simulink model "pidControl"  (R2019b)
settings: Solver=VariableStepAuto  StartTime=0.0  StopTime=10.0  RelTol=1e-3
undefined symbols (not defined in the file or in its folder): calib
libraries: arduinolib x10, simulink x4, dspstat3 x3
settings Model: Creator=Victor  LastModifiedBy=covasanvictor

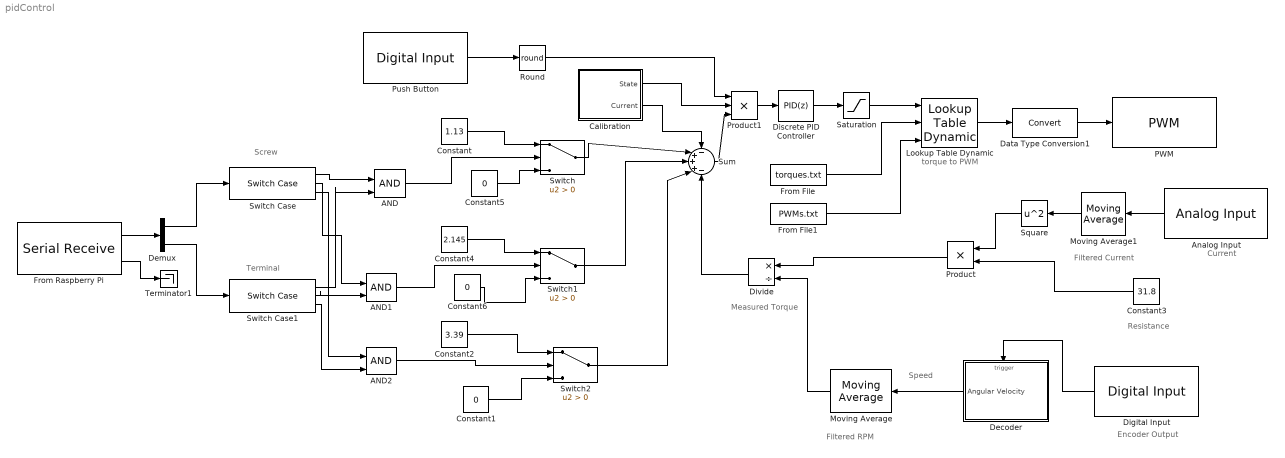
== system pidControl ==
  note: Filtered Current
  note: Filtered RPM
  note: Encoder Output
  note: Measured
      | Torque
  note: Speed
  note: Screw
  note: torque to PWM
  note: Current
  note: Resistance
  note: Terminal
  AND : Logic  IconShape=distinctive  AllPortsSameDT=off  OutDataTypeStr=boolean
  AND1 : Logic  IconShape=distinctive  AllPortsSameDT=off  OutDataTypeStr=boolean
  AND2 : Logic  IconShape=distinctive  AllPortsSameDT=off  OutDataTypeStr=boolean
  Analog Input : arduinolib/Analog Input  pinNumber=0  ReadResultsOnly=off  ConversionTriggerSource=Software  ExternalTriggerType=uint32( 0 )  OutputDataType=uint16  EnableConversionCompleteNotify=off  EnableOuputStatus=off  SampleTime=-1  blockPlatform=arduino
  "Calibration " : Subsystem
  Constant : Constant  Value=1.13
  Constant1 : Constant  Value=0
  Constant2 : Constant  Value=3.39
  Constant3 : Constant  Value=31.8
  Constant4 : Constant  Value=2.145
  Constant5 : Constant  Value=0
  Constant6 : Constant  Value=0
  Data Type Conversion1 : DataTypeConversion  OutMin=[0]  OutMax=[255]
  "Decoder " : Subsystem
  Demux : Demux  Outputs=2
  Digital Input : arduinolib/Digital Input  pinNumber=2  SampleTime=-1  blockPlatform=arduino
      settings: SourceProductName=Simulink Support Package for Arduino Hardware
  Discrete PID Controller : simulink/Continuous/PID Controller  Controller=PID  Form=Parallel  TimeDomain=Discrete-time  SampleTime=-1  IntegratorMethod=Forward Euler  FilterMethod=Forward Euler  ControllerParametersSource=internal  P=10  I=0.1  D=0  UseFilter=on  N=100  TunerSelectOption=Transfer Function Based (PID Tuner App)  InitialConditionSource=internal  InitialConditionForIntegrator=0  InitialConditionForFilter=0  DifferentiatorICPrevScaledInput=0  ExternalReset=none  TrackingMode=off  Kt=1  LimitOutput=off  UpperSaturationLimit=inf  LowerSaturationLimit=-inf  LinearizeAsGain=off  AntiWindupMode=none  Kb=1  POutMin=[]  POutMax=[]  IOutMin=[]  IOutMax=[]  DOutMin=[]  DOutMax=[]  NOutMin=[]  NOutMax=[]  SumOutMin=[]  SumOutMax=[]  SaturationOutMin=[]  SaturationOutMax=[]  PParamMin=[]  PParamMax=[]  IParamMin=[]  IParamMax=[]  DParamMin=[]  DParamMax=[]  NParamMin=[]  NParamMax=[]  KbParamMin=[]  KbParamMax=[]  KtParamMin=[]  KtParamMax=[]  KbOutMin=[]  KbOutMax=[]  KtOutMin=[]  KtOutMax=[]  IntegratorOutMin=[]  IntegratorOutMax=[]  FilterOutMin=[]  FilterOutMax=[]  SumI1OutMin=[]  SumI1OutMax=[]  SumI2OutMin=[]  SumI2OutMax=[]  SumI3OutMin=[]  SumI3OutMax=[]  SumI4OutMin=[]  SumI4OutMax=[]  SumDOutMin=[]  SumDOutMax=[]  DifferentiatorOutMin=[]  DifferentiatorOutMax=[]  FilterDiffOutCoefMin=[]  FilterDiffOutCoefMax=[]  ReciprocalOutMin=[]  ReciprocalOutMax=[]  SumDenOutMin=[]  SumDenOutMax=[]  SumNumOutMin=[]  SumNumOutMax=[]  DivideOutMin=[]  DivideOutMax=[]  IntegratorContinuousStateAttributes=''  IntegratorStateMustResolveToSignalObject=off  IntegratorRTWStateStorageClass=Auto  FilterContinuousStateAttributes=''  FilterStateMustResolveToSignalObject=off  FilterRTWStateStorageClass=Auto  ParallelPVariant=InternalParameters  IdealPVariant=Disabled  IVariant=InternalParameters  DVariant=InternalParameters  IntegratorVariant=Discrete  SatVariant=Disabled  AWVariant=Passthrough  PCopyVariant=Disabled  TRVariant=Disabled  FdbkBlocksVariant=Forward  IdealPFdbkVariant=Disabled  SatFdbkVariant=Disabled  DerivativeFilterVariant=ForwardEulerFilter  NVariant=InternalParameters  NCopyVariant=Disabled  FilterICVariant=InternalICsFilter  IntegratorICVariant=InternalICs  ExternalResetVariant=Disabled  TRSumVariant=Passthrough  SumFdbkVariant=Disabled  SumVariant=Sum_PID
  Divide : Product  Inputs=*/
  From File : FromFile  FileName=torques.txt  SampleTime=0
  From File1 : FromFile  FileName=PWMs.txt  SampleTime=0
  "From Raspberry Pi " : arduinolib/Serial Receive  isARMArch=off  portNumber=0  DataType=uint8  Datalength=2  SampleTime=0.1  showOutStatus=on  blockPlatform=arduino
      settings: SourceProductName=Simulink Support Package for Arduino Hardware  SourceProductBaseCode=ARDUINO
  Lookup Table Dynamic : simulink/Lookup Tables/Lookup Table Dynamic  LookUpMeth=Interpolation-Use End Values  OutDataType=fixdt('double')  OutScaling=[]  OutputDataTypeScalingMode=Specify via dialog  OutDataTypeStr=double  DoSatur=off
  Moving Average : dspstat3/Moving Average  Method=Sliding window  ForgettingFactorPort=off  SpecifyWindowLength=on  WindowLength=4  ForgettingFactor=0.9  SimulateUsing=Code generation
  Moving Average1 : dspstat3/Moving Average  Method=Sliding window  ForgettingFactorPort=off  SpecifyWindowLength=on  WindowLength=4  ForgettingFactor=0.9  SimulateUsing=Code generation
  PWM : arduinolib/PWM  pinNumber=6  EnableInputFrequency=off  InitialFrequency=2000  InitialDutyCycle=0  NotificationType=None  blockPlatform=arduino
  Product : Product
  Product1 : Product  Inputs=3
  "Push Button " : arduinolib/Digital Input  pinNumber=8  SampleTime=-1  blockPlatform=arduino
      settings: SourceProductName=Simulink Support Package for Arduino Hardware
  Round : Rounding  Operator=round
  Saturation : Saturate
  Square : Math  Operator=square  SignedPower=off  SaturateOnIntegerOverflow=on
  Sum : Sum  Inputs=-+++-
  Switch : Switch  Criteria=u2 > Threshold
  Switch Case : SwitchCase  CaseConditions={1, 2, 3}  ShowDefaultCase=off
  Switch Case1 : SwitchCase  CaseConditions={1, 2, 3}  ShowDefaultCase=off
  Switch1 : Switch  Criteria=u2 > Threshold
  Switch2 : Switch  Criteria=u2 > Threshold
  Terminator1 : Terminator
  wires:
  Constant3/1 -> Product/2
  Square/1 -> Product/1
  "Decoder "/1("Angular Velocity ") -> Moving Average/1
  Product/1 -> Divide/1
  Discrete PID Controller/1 -> Saturation/1
  Constant/1 -> Switch/1
  Saturation/1 -> Lookup Table Dynamic/1
  From File/1 -> Lookup Table Dynamic/2
  From File1/1 -> Lookup Table Dynamic/3
  Switch Case/1 -> AND/1
  Switch Case1/1 -> AND/2
  AND/1 -> Switch/2
  Moving Average/1 -> Divide/2
  Constant5/1 -> Switch/3
  Switch Case1/2 -> AND1/2
  Switch Case/2 -> AND1/1
  Constant6/1 -> Switch1/3
  Constant4/1 -> Switch1/1
  AND1/1 -> Switch1/2
  Switch Case/3 -> AND2/1
  Switch Case1/3 -> AND2/2
  Constant1/1 -> Switch2/3
  Constant2/1 -> Switch2/1
  AND2/1 -> Switch2/2
  "From Raspberry Pi "/1 -> Demux/1
  Demux/1 -> Switch Case/1
  Demux/2 -> Switch Case1/1
  "From Raspberry Pi "/2 -> Terminator1/1
  Lookup Table Dynamic/1 -> Data Type Conversion1/1
  Data Type Conversion1/1 -> PWM/1
  Digital Input/1 -> "Decoder "/Trigger
  Product1/1 -> Discrete PID Controller/1
  "Calibration "/1(State) -> Product1/2
  Sum/1 -> Product1/3
  "Push Button "/1 -> Round/1
  Round/1 -> Product1/1
  Divide/1 -> Sum/5
  Switch2/1 -> Sum/4
  Switch1/1 -> Sum/3
  Switch/1 -> Sum/2
  "Calibration "/2("Current ") -> Sum/1
  Moving Average1/1 -> Square/1
  Analog Input/1 -> Moving Average1/1

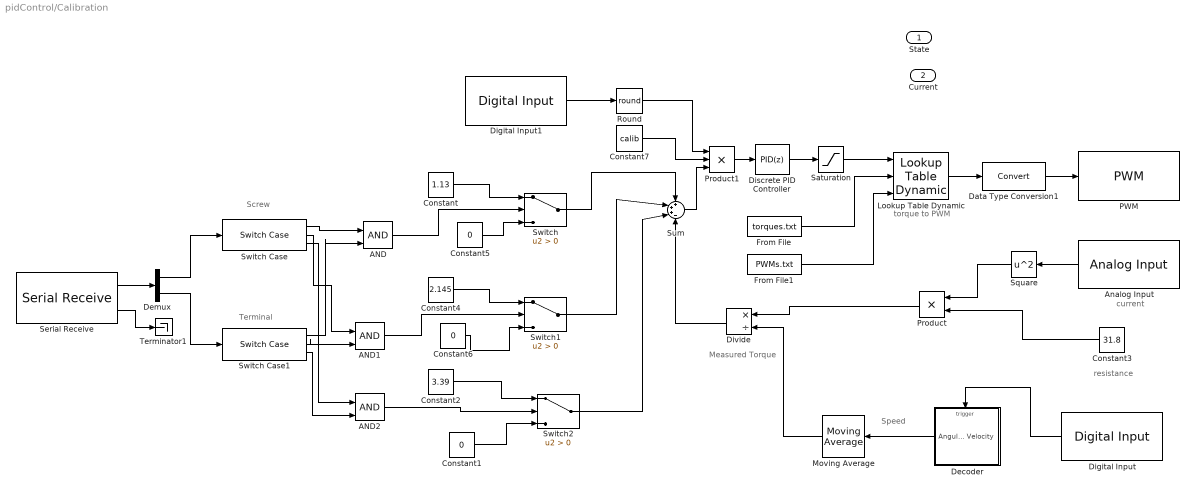
== system pidControl/Calibration  ==
  note: Terminal
  note: current
  note: resistance
  note: Screw
  note: torque to PWM
  note: Speed
  note: Measured
      | Torque
  AND : Logic  IconShape=distinctive  AllPortsSameDT=off  OutDataTypeStr=boolean
  AND1 : Logic  IconShape=distinctive  AllPortsSameDT=off  OutDataTypeStr=boolean
  AND2 : Logic  IconShape=distinctive  AllPortsSameDT=off  OutDataTypeStr=boolean
  Analog Input : arduinolib/Analog Input  pinNumber=0  ReadResultsOnly=off  ConversionTriggerSource=Software  ExternalTriggerType=uint32( 0 )  OutputDataType=uint16  EnableConversionCompleteNotify=off  EnableOuputStatus=off  SampleTime=-1  blockPlatform=arduino
  Constant : Constant  Value=1.13
  Constant1 : Constant  Value=0
  Constant2 : Constant  Value=3.39
  Constant3 : Constant  Value=31.8
  Constant4 : Constant  Value=2.145
  Constant5 : Constant  Value=0
  Constant6 : Constant  Value=0
  Constant7 : Constant  Value=calib
  Data Type Conversion1 : DataTypeConversion  OutMin=[0]  OutMax=[255]
  "Decoder " : Subsystem
  Demux : Demux  Outputs=2
  Digital Input : arduinolib/Digital Input  pinNumber=2  SampleTime=-1  blockPlatform=arduino
      settings: SourceProductName=Simulink Support Package for Arduino Hardware
  Digital Input1 : arduinolib/Digital Input  pinNumber=8  SampleTime=-1  blockPlatform=arduino
      settings: SourceProductName=Simulink Support Package for Arduino Hardware
  Discrete PID Controller : simulink/Continuous/PID Controller  Controller=PID  Form=Parallel  TimeDomain=Discrete-time  SampleTime=-1  IntegratorMethod=Forward Euler  FilterMethod=Forward Euler  ControllerParametersSource=internal  P=10  I=0.1  D=0  UseFilter=on  N=100  TunerSelectOption=Transfer Function Based (PID Tuner App)  InitialConditionSource=internal  InitialConditionForIntegrator=0  InitialConditionForFilter=0  DifferentiatorICPrevScaledInput=0  ExternalReset=none  TrackingMode=off  Kt=1  LimitOutput=off  UpperSaturationLimit=inf  LowerSaturationLimit=-inf  LinearizeAsGain=off  AntiWindupMode=none  Kb=1  POutMin=[]  POutMax=[]  IOutMin=[]  IOutMax=[]  DOutMin=[]  DOutMax=[]  NOutMin=[]  NOutMax=[]  SumOutMin=[]  SumOutMax=[]  SaturationOutMin=[]  SaturationOutMax=[]  PParamMin=[]  PParamMax=[]  IParamMin=[]  IParamMax=[]  DParamMin=[]  DParamMax=[]  NParamMin=[]  NParamMax=[]  KbParamMin=[]  KbParamMax=[]  KtParamMin=[]  KtParamMax=[]  KbOutMin=[]  KbOutMax=[]  KtOutMin=[]  KtOutMax=[]  IntegratorOutMin=[]  IntegratorOutMax=[]  FilterOutMin=[]  FilterOutMax=[]  SumI1OutMin=[]  SumI1OutMax=[]  SumI2OutMin=[]  SumI2OutMax=[]  SumI3OutMin=[]  SumI3OutMax=[]  SumI4OutMin=[]  SumI4OutMax=[]  SumDOutMin=[]  SumDOutMax=[]  DifferentiatorOutMin=[]  DifferentiatorOutMax=[]  FilterDiffOutCoefMin=[]  FilterDiffOutCoefMax=[]  ReciprocalOutMin=[]  ReciprocalOutMax=[]  SumDenOutMin=[]  SumDenOutMax=[]  SumNumOutMin=[]  SumNumOutMax=[]  DivideOutMin=[]  DivideOutMax=[]  IntegratorContinuousStateAttributes=''  IntegratorStateMustResolveToSignalObject=off  IntegratorRTWStateStorageClass=Auto  FilterContinuousStateAttributes=''  FilterStateMustResolveToSignalObject=off  FilterRTWStateStorageClass=Auto  ParallelPVariant=InternalParameters  IdealPVariant=Disabled  IVariant=InternalParameters  DVariant=InternalParameters  IntegratorVariant=Discrete  SatVariant=Disabled  AWVariant=Passthrough  PCopyVariant=Disabled  TRVariant=Disabled  FdbkBlocksVariant=Forward  IdealPFdbkVariant=Disabled  SatFdbkVariant=Disabled  DerivativeFilterVariant=ForwardEulerFilter  NVariant=InternalParameters  NCopyVariant=Disabled  FilterICVariant=InternalICsFilter  IntegratorICVariant=InternalICs  ExternalResetVariant=Disabled  TRSumVariant=Passthrough  SumFdbkVariant=Disabled  SumVariant=Sum_PID
  Divide : Product  Inputs=*/
  From File : FromFile  FileName=torques.txt  SampleTime=0
  From File1 : FromFile  FileName=PWMs.txt  SampleTime=0
  Lookup Table Dynamic : simulink/Lookup Tables/Lookup Table Dynamic  LookUpMeth=Interpolation-Use End Values  OutDataType=fixdt('double')  OutScaling=[]  OutputDataTypeScalingMode=Specify via dialog  OutDataTypeStr=double  DoSatur=off
  Moving Average : dspstat3/Moving Average  Method=Sliding window  ForgettingFactorPort=off  SpecifyWindowLength=on  WindowLength=4  ForgettingFactor=0.9  SimulateUsing=Code generation
  PWM : arduinolib/PWM  pinNumber=6  EnableInputFrequency=off  InitialFrequency=2000  InitialDutyCycle=0  NotificationType=None  blockPlatform=arduino
  Product : Product
  Product1 : Product  Inputs=3
  Round : Rounding  Operator=round
  Saturation : Saturate
  Serial Receive : arduinolib/Serial Receive  isARMArch=off  portNumber=0  DataType=uint8  Datalength=2  SampleTime=0.1  showOutStatus=on  blockPlatform=arduino
      settings: SourceProductName=Simulink Support Package for Arduino Hardware  SourceProductBaseCode=ARDUINO
  Square : Math  Operator=square  SignedPower=off  SaturateOnIntegerOverflow=on
  Sum : Sum  Inputs=+++-
  Switch : Switch  Criteria=u2 > Threshold
  Switch Case : SwitchCase  CaseConditions={1, 2, 3}  ShowDefaultCase=off
  Switch Case1 : SwitchCase  CaseConditions={1, 2, 3}  ShowDefaultCase=off
  Switch1 : Switch  Criteria=u2 > Threshold
  Switch2 : Switch  Criteria=u2 > Threshold
  Terminator1 : Terminator
  State : Outport
  "Current " : Outport  Port=2
  wires:
  Data Type Conversion1/1 -> PWM/1
  Product1/1 -> Discrete PID Controller/1
  Sum/1 -> Product1/3
  Analog Input/1 -> Square/1
  AND2/1 -> Switch2/2
  "Decoder "/1("Angular Velocity ") -> Moving Average/1
  Lookup Table Dynamic/1 -> Data Type Conversion1/1
  Digital Input1/1 -> Round/1
  Switch/1 -> Sum/1
  Serial Receive/2 -> Terminator1/1
  From File1/1 -> Lookup Table Dynamic/3
  Demux/1 -> Switch Case/1
  Square/1 -> Product/1
  Switch Case/3 -> AND2/1
  Constant1/1 -> Switch2/3
  AND1/1 -> Switch1/2
  AND/1 -> Switch/2
  Switch Case1/1 -> AND/2
  Constant7/1 -> Product1/2
  Round/1 -> Product1/1
  Discrete PID Controller/1 -> Saturation/1
  Constant/1 -> Switch/1
  Constant5/1 -> Switch/3
  Switch2/1 -> Sum/3
  Digital Input/1 -> "Decoder "/Trigger
  Saturation/1 -> Lookup Table Dynamic/1
  Switch Case/1 -> AND/1
  Switch Case1/3 -> AND2/2
  Moving Average/1 -> Divide/2
  Demux/2 -> Switch Case1/1
  Constant3/1 -> Product/2
  Constant4/1 -> Switch1/1
  Switch1/1 -> Sum/2
  Divide/1 -> Sum/4
  Constant2/1 -> Switch2/1
  Constant6/1 -> Switch1/3
  Product/1 -> Divide/1
  Switch Case1/2 -> AND1/2
  Serial Receive/1 -> Demux/1
  From File/1 -> Lookup Table Dynamic/2
  Switch Case/2 -> AND1/1

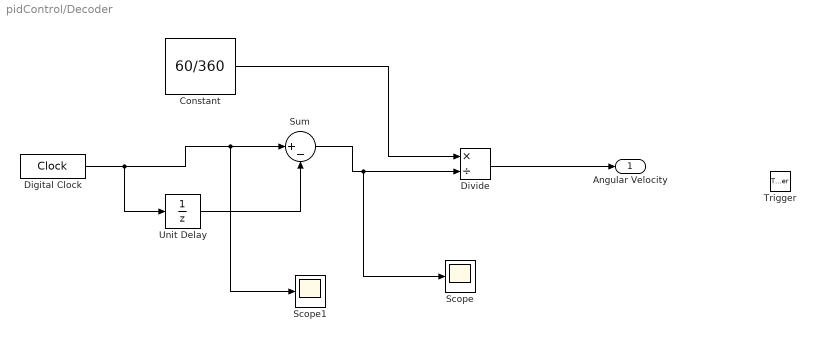
== system pidControl/Decoder  ==
  Trigger : TriggerPort  TriggerType=either  VariantControl=Variant  OutputDataType=double  PortDimensions=1
  Constant : Constant  Value=60/360  SampleTime=-1
  Digital Clock : DigitalClock  SampleTime=-1
  Divide : Product  Inputs=*/
  Scope : Scope
  Scope1 : Scope
  Sum : Sum  Inputs=|+-
  Unit Delay : UnitDelay  SampleTime=-1  HasFrameUpgradeWarning=on
  "Angular Velocity " : Outport  VectorParamsAs1DForOutWhenUnconnected=off
  wires:
  Unit Delay/1 -> Sum/2
  Digital Clock/1 -> Unit Delay/1, Scope1/1, Sum/1
  Divide/1 -> "Angular Velocity "/1
  Constant/1 -> Divide/1
  Sum/1 -> Scope/1, Divide/2

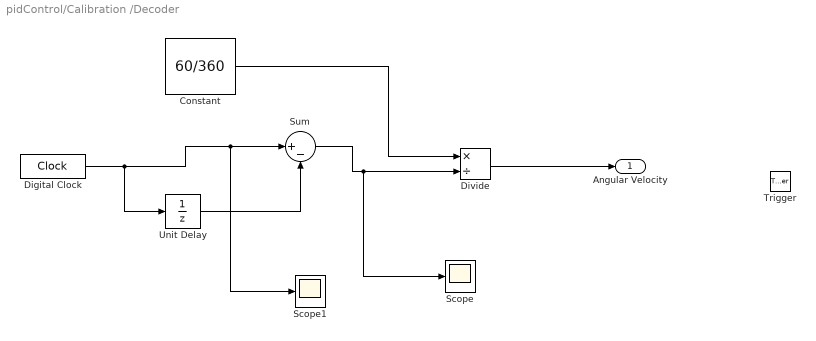
== system pidControl/Calibration /Decoder  ==
  Trigger : TriggerPort  TriggerType=either  VariantControl=Variant  OutputDataType=double  PortDimensions=1
  Constant : Constant  Value=60/360  SampleTime=-1
  Digital Clock : DigitalClock  SampleTime=-1
  Divide : Product  Inputs=*/
  Scope : Scope
  Scope1 : Scope
  Sum : Sum  Inputs=|+-
  Unit Delay : UnitDelay  SampleTime=-1  HasFrameUpgradeWarning=on
  "Angular Velocity " : Outport  VectorParamsAs1DForOutWhenUnconnected=off
  wires:
  Unit Delay/1 -> Sum/2
  Digital Clock/1 -> Unit Delay/1, Scope1/1, Sum/1
  Divide/1 -> "Angular Velocity "/1
  Constant/1 -> Divide/1
  Sum/1 -> Scope/1, Divide/2
